simulink model "lstm_train_data"  (R2024b)
settings: Solver=ode45  StartTime=0.0  StopTime=120000  RelTol=1e-3
settings Model: Creator=User  LastModifiedBy=HP
settings SolverCC: AlgebraicLoopSolver=TrustRegion
settings DebuggingCC: UnconnectedInputMsg=warning  UnconnectedOutputMsg=warning  UnconnectedLineMsg=warning  ArithmeticOperatorsInVariantConditions=warning
settings ModelReferenceCC: EnableRefExpFcnMdlSchedulingChecks=on
settings SFSimCC: CustomCodeUndefinedFunction=UseInterfaceOnly
settings RTWCC: GPUComputeCapability=3.5

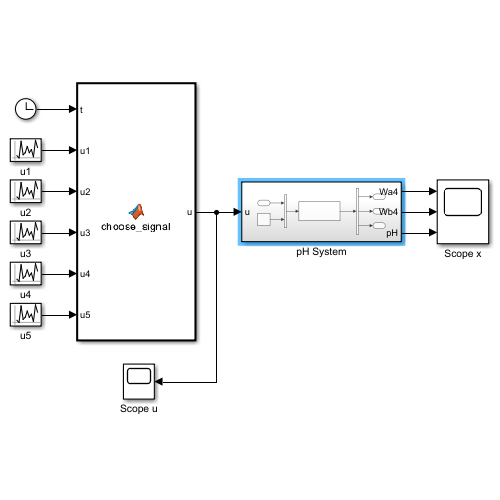
[thumbnail: Simulink's stored preview of the top-level diagram]
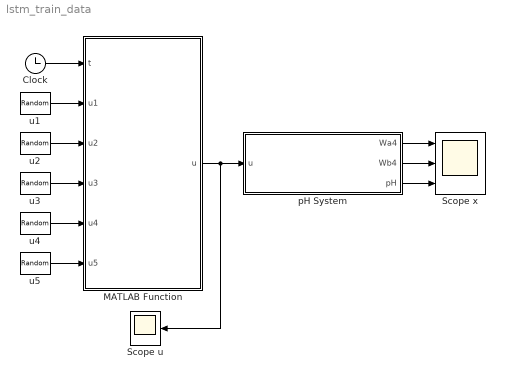
== system lstm_train_data ==
  " pH System " : Subsystem
  Clock : Clock
  MATLAB Function : MATLAB Function  TreatAsAtomicUnit=on
  Scope u : Scope
  Scope x : Scope  NumInputPorts=3
  u1 : UniformRandomNumber  Minimum=0  Maximum=50  Seed=1  SampleTime=300
  u2 : UniformRandomNumber  Minimum=0  Maximum=50  Seed=1  SampleTime=150
  u3 : UniformRandomNumber  Minimum=0  Maximum=50  Seed=1  SampleTime=75
  u4 : UniformRandomNumber  Minimum=0  Maximum=50  Seed=1  SampleTime=20
  u5 : UniformRandomNumber  Minimum=0  Maximum=50  Seed=1  SampleTime=5
  wires:
  " pH System "/1(Wa4) -> Scope x/1
  " pH System "/2(Wb4) -> Scope x/2
  " pH System "/3(pH) -> Scope x/3
  u1/1 -> MATLAB Function/2(u1)
  u2/1 -> MATLAB Function/3(u2)
  u3/1 -> MATLAB Function/4(u3)
  u4/1 -> MATLAB Function/5(u4)
  u5/1 -> MATLAB Function/6(u5)
  Clock/1 -> MATLAB Function/1(t)
  MATLAB Function/1(u) -> " pH System "/1(u), Scope u/1

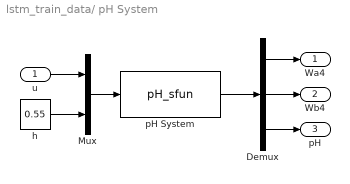
== system lstm_train_data/ pH System  ==
  u : Inport
  " h " : Constant  Value=0.55
  Demux : Demux  Outputs=3
  Mux : Mux  Inputs=2
  pH System : S-Function  FunctionName=pH_sfun  SFunctionDeploymentMode=off  EnableBusSupport=off
  Wa4 : Outport  VectorParamsAs1DForOutWhenUnconnected=off
  Wb4 : Outport  Port=2  VectorParamsAs1DForOutWhenUnconnected=off
  pH : Outport  Port=3  VectorParamsAs1DForOutWhenUnconnected=off
  wires:
  Mux/1 -> pH System/1
  pH System/1 -> Demux/1
  u/1 -> Mux/1
  Demux/2 -> Wb4/1
  Demux/1 -> Wa4/1
  Demux/3 -> pH/1
  " h "/1 -> Mux/2

== matlab function lstm_train_data/MATLAB Function ==
  data: t input; u output; u1 input; u2 input; u3 input; u4 input; u5 input
function u = choose_signal(t,u1,u2,u3,u4,u5)
u_opts = [u1,u2,u3,u4,u5];
sim_time = 120000;
stops = 0:round(sim_time/numel(u_opts)):sim_time;
u = u_opts(1);
for i = 1:numel(stops)-1
    if (t >= stops(i)) && (t <= stops(i+1))
        u = u_opts(i);
        break;
    end
end
